simulink model "KF3_to_play_with_real"  (R2019b)
settings: Solver=ode3  StartTime=0.0  StopTime=10.0  FixedStep=0.0001  MaxStep=.001  RelTol=1e-3
values from neighbouring files (symbols this model uses):
  Fes = F-L*H    [KF3_Script.m]    (also in KF_Script.m; LQG_Script.m)
  L = (dlqr(F',H',Q,R))'    [KF3_Script.m]    (also in KF_Script.m; LQG_Script.m)
undefined symbols (not defined in the file or in its folder): G
settings Model: Creator=oboe  LastModifiedBy=Luca
settings DataIOCC: LimitDataPoints=on  SaveFormat=Array  ReturnWorkspaceOutputs=off
settings OptimizationCC: LifeSpan=inf
settings DebuggingCC: SolverPrmCheckMsg=warning  SFUnexpectedBacktrackingDiag=warning  SFNoUnconditionalDefaultTransitionDiag=warning  SFExecutionAtInitializationDiag=none  ArithmeticOperatorsInVariantConditions=warning
settings HardwareCC: ProdBitPerPointer=32  ProdBitPerSizeT=32  ProdBitPerPtrDiffT=32  ProdLargestAtomicFloat=None  ProdIntDivRoundTo=Undefined  ProdEndianess=Unspecified  ProdWordSize=32  ProdHWDeviceType=32-bit Generic
settings ModelReferenceCC: PropagateSignalLabelsOutOfModel=off
settings SFSimCC: SimUseLocalCustomCode=off  CustomCodeUndefinedFunction=UseInterfaceOnly
settings RTWCC: RTWUseLocalCustomCode=off
settings CodeAppCC: StateflowObjectComments=on
settings GRTTargetCC: TargetLangStandard=C89/C90 (ANSI)
settings ConfigComp: CovMetricSettings=dw  CovHtmlReporting=on  CovSaveCumulativeToWorkspaceVar=on  CovSaveSingleToWorkspaceVar=on  CovExternalEMLEnable=off  CovSFcnEnable=off

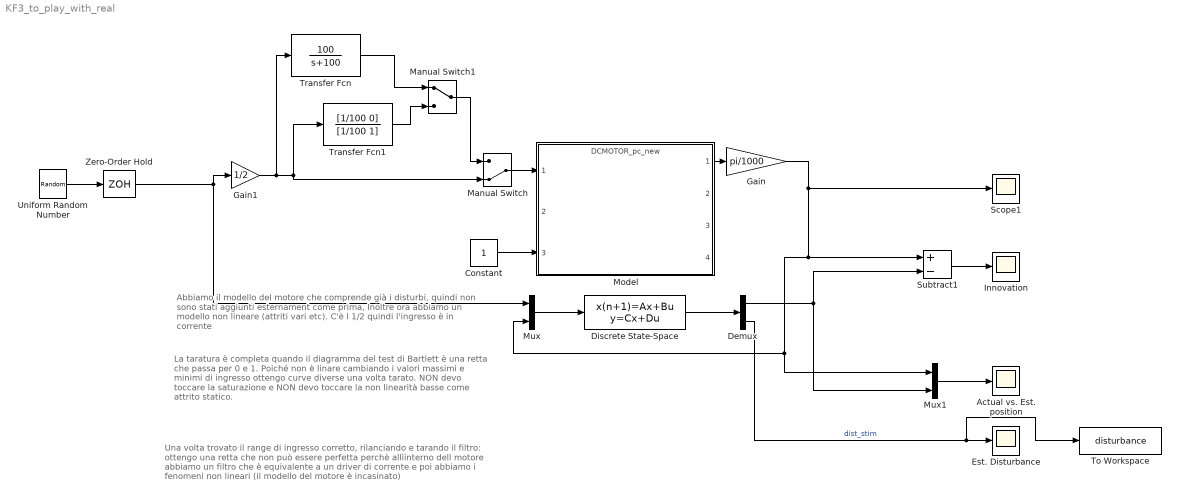
== system KF3_to_play_with_real ==
  note: Abbiamo il modello del motore che comprende già i disturbi, quindi non sono stati aggiunti esternament come prima, Inoltre ora
      | abbiamo un modello non lineare (attriti vari etc). C'è l 1/2 quindi l'ingresso è in corrente
  note: Una volta trovato il range di ingresso corretto, rilanciando
      | e tarando il filtro: ottengo una retta che non può essere
      | perfetta perchè allìinterno dell motore abbiamo un filtro che
      | è equivalente a un driver di corrente e poi abbiamo i fenomeni
      | non lineari (il modello del motore è incasinato)
  note: La taratura è completa quando il diagramma del test di
      | Bartlett è una retta che passa per 0 e 1. Poiché non è
      | linare cambiando i valori massimi e minimi di ingresso
      | ottengo curve diverse una volta tarato. NON devo toccare
      | la saturazione e NON devo toccare la non linearità basse
      | come attrito statico.
  Actual vs. Est. position : Scope
  Constant : Constant
  Demux : Demux  Outputs=3
  Discrete State-Space : DiscreteStateSpace  A=Fes  B=[G L]  C=eye(3)  D=zeros(3,2)  SampleTime=.001
  Est. Disturbance : Scope
  Gain : Gain  Gain=pi/1000
  Gain1 : Gain  Gain=1/2
  Innovation : Scope
  Manual Switch : ManualSwitch  CurrentSetting=0
  Manual Switch1 : ManualSwitch
  Model : ModelReference  ModelNameDialog=DCMOTOR_pc_new.slxp  ModelReferenceVersion=1.21  CopyOfModelProtected=on
  Mux : Mux  Inputs=2
  Mux1 : Mux  Inputs=2
  Scope1 : Scope
  Subtract1 : Sum  Inputs=+-
  To Workspace : ToWorkspace  VariableName=disturbance  SaveFormat=Timeseries  SampleTime=-1
  Transfer Fcn : TransferFcn  Numerator=[100]  Denominator=[1 100]
  Transfer Fcn1 : TransferFcn  Numerator=[1/100 0]  Denominator=[1/100 1]
  Uniform Random Number : UniformRandomNumber  Minimum=-2  Maximum=2  SampleTime=0.001
  Zero-Order Hold : ZeroOrderHold  SampleTime=0.001
  wires:
  Mux/1 -> Discrete State-Space/1
  Discrete State-Space/1 -> Demux/1
  Demux/1 -> Mux1/2, Subtract1/2
  Mux1/1 -> Actual vs. Est. position/1
  Subtract1/1 -> Innovation/1
  Gain/1 -> Mux/2, Mux1/1, Subtract1/1, Scope1/1
  Zero-Order Hold/1 -> Gain1/1, Mux/1
  Uniform Random Number/1 -> Zero-Order Hold/1
  Demux/3 -> To Workspace/1, Est. Disturbance/1  "dist_stim"
  Model/1 -> Gain/1
  Constant/1 -> Model/3
  Gain1/1 -> Transfer Fcn/1, Transfer Fcn1/1, Manual Switch/2
  Transfer Fcn/1 -> Manual Switch1/1
  Transfer Fcn1/1 -> Manual Switch1/2
  Manual Switch/1 -> Model/1
  Manual Switch1/1 -> Manual Switch/1
